simulink model "Control_Block_step"  (R2020a)
settings: Solver=VariableStepAuto  StartTime=0.0  StopTime=10.0  RelTol=1e-3
libraries: fuzblock x1
settings Model: Creator=chris  LastModifiedBy=chris

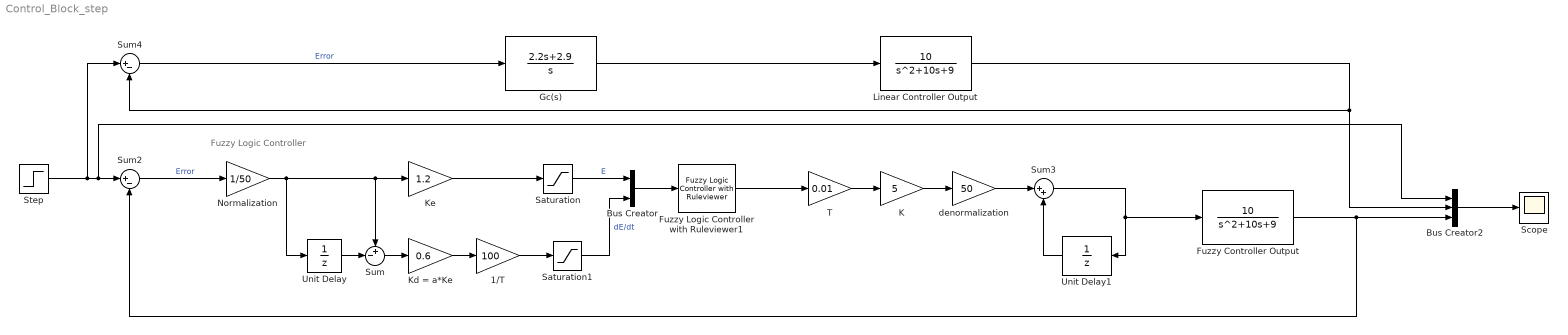
== system Control_Block_step ==
  note: Fuzzy Logic Controller
  1/T : Gain  Gain=100
  Bus Creator : BusCreator  Inputs=2
  Bus Creator2 : BusCreator  Inputs=3
  Fuzzy Controller Output : TransferFcn  Numerator=[10]  Denominator=[1 10 9]
  Fuzzy Logic Controller with Ruleviewer1 : fuzblock/Fuzzy Logic  Controller  with Ruleviewer  fismatrix=FLC  Ts=0.01
  Gc(s) : TransferFcn  Numerator=[0 2.2 2.9]  Denominator=[1 0]
  K : Gain  Gain=5
  Kd = a*Ke : Gain  Gain=0.6
  Ke : Gain  Gain=1.2
  Linear Controller Output : TransferFcn  Numerator=[10]  Denominator=[1 10 9]
  Normalization : Gain  Gain=1/50
  Saturation : Saturate  UpperLimit=1  LowerLimit=-1
  Saturation1 : Saturate  UpperLimit=1  LowerLimit=-1
  Scope : Scope
  Step : Step  Time=0  After=50  SampleTime=0.01
  Sum : Sum  Inputs=+-|
  Sum2 : Sum  Inputs=|+-
  Sum3 : Sum  Inputs=|++
  Sum4 : Sum  Inputs=|+-
  T : Gain  Gain=0.01
  Unit Delay : UnitDelay  SampleTime=-1  HasFrameUpgradeWarning=on
  Unit Delay1 : UnitDelay  SampleTime=-1  HasFrameUpgradeWarning=on
  denormalization : Gain  Gain=50
  wires:
  Step/1 -> Sum4/1, Bus Creator2/1, Sum2/1
  Sum3/1 -> Unit Delay1/1, Fuzzy Controller Output/1
  Fuzzy Controller Output/1 -> Bus Creator2/3, Sum2/2
  Sum2/1 -> Normalization/1  "Error"
  1/T/1 -> Saturation1/1
  K/1 -> denormalization/1
  Unit Delay1/1 -> Sum3/2
  Saturation/1 -> Bus Creator/1  "E"
  Sum/1 -> Kd = a*Ke/1
  Unit Delay/1 -> Sum/2
  denormalization/1 -> Sum3/1
  Kd = a*Ke/1 -> 1/T/1
  Saturation1/1 -> Bus Creator/2  "dE/dt"
  T/1 -> K/1
  Ke/1 -> Saturation/1
  Normalization/1 -> Unit Delay/1, Sum/1, Ke/1
  Fuzzy Logic Controller with Ruleviewer1/1 -> T/1
  Bus Creator/1 -> Fuzzy Logic Controller with Ruleviewer1/1
  Linear Controller Output/1 -> Bus Creator2/2, Sum4/2
  Gc(s)/1 -> Linear Controller Output/1
  Sum4/1 -> Gc(s)/1  "Error"
  Bus Creator2/1 -> Scope/1
